simulink model "statefeedback"  (R2019b)
settings: Solver=VariableStepAuto  StartTime=0.0  StopTime=2  RelTol=1e-3
values from neighbouring files (symbols this model uses):
  A11 = A(1,1)    [lqrfeedback_params.m]    (also in observerbasednonlin_params.m = Ao(1,1); observerdesign_params.m; statefeedback_params.m)
  A12 = A(1,2)    [lqrfeedback_params.m]    (also in observerbasednonlin_params.m = Ao(1,2); observerdesign_params.m; statefeedback_params.m)
  A21 = A(2,1)    [lqrfeedback_params.m]    (also in observerbasednonlin_params.m = Ao(2,1); observerdesign_params.m; statefeedback_params.m)
  A22 = A(2,2)    [lqrfeedback_params.m]    (also in observerbasednonlin_params.m = Ao(2,2); observerdesign_params.m; statefeedback_params.m)
  B1 = B(1)    [lqrfeedback_params.m]    (also in observerbasednonlin_params.m; observerdesign_params.m; statefeedback_params.m)
  h1eq = 0    [lqrfeedback_params.m]    (also in observerbasednonlin_params.m; observerdesign_params.m; statefeedback_params.m; statefeedbacknonlin_params.m)
  h2eq = 0    [lqrfeedback_params.m]    (also in observerbasednonlin_params.m; observerdesign_params.m; statefeedback_params.m; statefeedbacknonlin_params.m)
  k1 = k(1)    [lqrfeedback_params.m]    (also in observerbasednonlin_params.m = 1.095; observerdesign_params.m = 0.0151; statefeedback_params.m = 1.09; statefeedbacknonlin_params.m = 1.09)
  k2 = k(2)    [lqrfeedback_params.m]    (also in observerbasednonlin_params.m = 87.12; observerdesign_params.m = 0.3997; statefeedback_params.m = 86.1515; statefeedbacknonlin_params.m = 86.1515)
  qeq = 0    [lqrfeedback_params.m]    (also in observerbasednonlin_params.m; observerdesign_params.m; statefeedback_params.m)
settings Model: Creator=SAI JOSHITHA  LastModifiedBy=SAI JOSHITHA

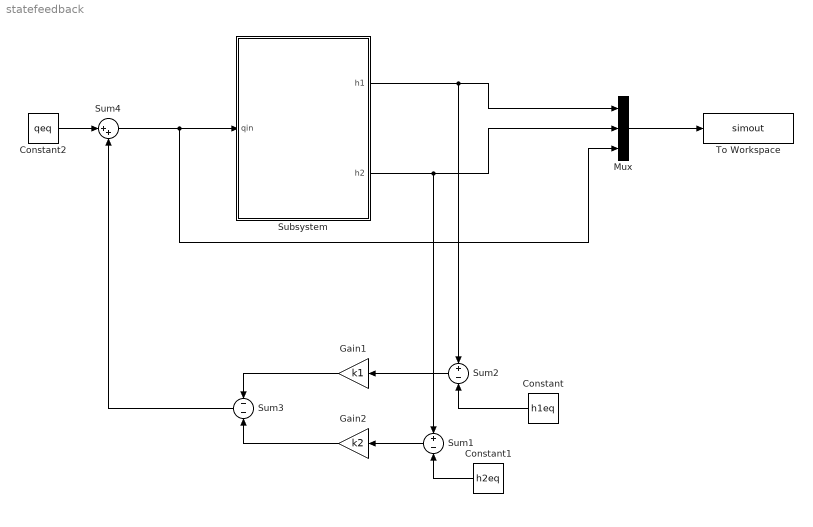
== system statefeedback ==
  Constant : Constant  Value=h1eq
  Constant1 : Constant  Value=h2eq
  Constant2 : Constant  Value=qeq
  Gain1 : Gain  Gain=k1
  Gain2 : Gain  Gain=k2
  Mux : Mux  Inputs=3
  Subsystem : Subsystem
  Sum1 : Sum  Inputs=+-
  Sum2 : Sum  Inputs=+-
  Sum3 : Sum  Inputs=--
  Sum4 : Sum  Inputs=|++
  To Workspace : ToWorkspace  VariableName=simout  SaveFormat=Timeseries  SampleTime=-1
  wires:
  Mux/1 -> To Workspace/1
  Subsystem/1(h1) -> Sum2/1, Mux/1
  Subsystem/2(h2) -> Sum1/1, Mux/2
  Constant1/1 -> Sum1/2
  Sum2/1 -> Gain1/1
  Sum1/1 -> Gain2/1
  Gain1/1 -> Sum3/1
  Constant/1 -> Sum2/2
  Gain2/1 -> Sum3/2
  Sum4/1 -> Mux/3, Subsystem/1(qin)
  Sum3/1 -> Sum4/2
  Constant2/1 -> Sum4/1

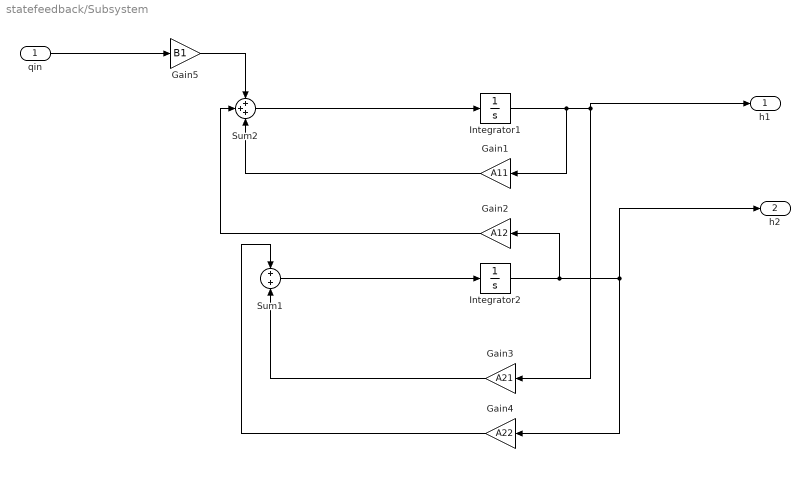
== system statefeedback/Subsystem ==
  qin : Inport
  Gain1 : Gain  Gain=A11
  Gain2 : Gain  Gain=A12
  Gain3 : Gain  Gain=A21
  Gain4 : Gain  Gain=A22
  Gain5 : Gain  Gain=B1
  Integrator1 : Integrator  InitialCondition=1
  Integrator2 : Integrator  InitialCondition=1
  Sum1 : Sum
  Sum2 : Sum  Inputs=+++
  h1 : Outport
  h2 : Outport  Port=2
  wires:
  Integrator2/1 -> Gain2/1, h2/1, Gain4/1
  Integrator1/1 -> Gain1/1, Gain3/1, h1/1
  Gain3/1 -> Sum1/2
  Sum2/1 -> Integrator1/1
  Gain4/1 -> Sum1/1
  Gain2/1 -> Sum2/2
  Gain5/1 -> Sum2/1
  Sum1/1 -> Integrator2/1
  Gain1/1 -> Sum2/3
  qin/1 -> Gain5/1
